simulink model "ej1"  (R2013a)
settings: Solver=ode45  StartTime=0.0  StopTime=(N-1)/Fs  MaxStep=1/Fs  MinStep=1/Fs  RelTol=1/Fs  AbsTol=1/Fs
settings Model: Creator=nazaretrogue  LastModifiedBy=nazaretrogue
settings SolverCC: InitialStep=1/Fs

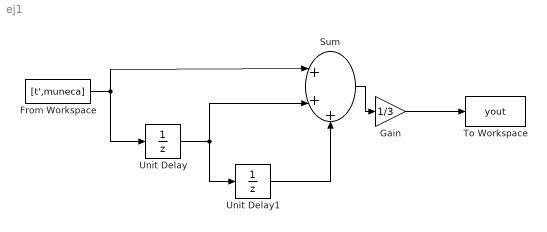
== system ej1 ==
  From Workspace : FromWorkspace  VariableName=[t',muneca]  SampleTime=0
  Gain : Gain  Gain=1/3
  Sum : Sum  Inputs=|+++
  To Workspace : ToWorkspace  VariableName=yout  SampleTime=-1
      settings: MaxDataPoints=N
  Unit Delay : UnitDelay  SampleTime=-1
  Unit Delay1 : UnitDelay  SampleTime=-1
  wires:
  From Workspace/1 -> Unit Delay/1, Sum/1
  Unit Delay/1 -> Sum/2, Unit Delay1/1
  Unit Delay1/1 -> Sum/3
  Sum/1 -> Gain/1
  Gain/1 -> To Workspace/1
